simulink model "Longitudinal_Simulink_MaskedParameter_WithOutput_Stateflow"  (Simulink 7.1)
settings: Solver=ode45  StartTime=0.0  StopTime=2.0  RelTol=1e-3
settings Model: Creator=Meisel  LastModifiedBy=Meisel

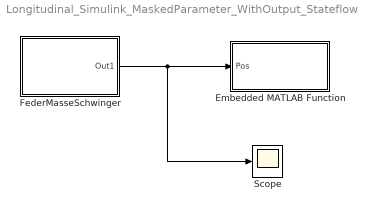
== system Longitudinal_Simulink_MaskedParameter_WithOutput_Stateflow ==
  Embedded MATLAB Function : Stateflow chart
  FederMasseSchwinger : Subsystem  mask{k_init=1000, m=1, l0=1}
      mask prompts: k_init "Federkonstanten"; m "Massen"; l0 "Federlänge"
  Scope : Scope
      settings: TimeRange=0.1792929292929293  YMin=1  YMax=1.888157894736842
  wires:
  FederMasseSchwinger/1(Out1) -> Embedded MATLAB Function/1(Pos), Scope/1

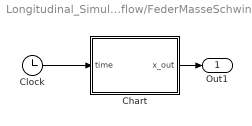
== system Longitudinal_Simulink_MaskedParameter_WithOutput_Stateflow/FederMasseSchwinger ==
  Chart : Stateflow chart
  Clock : Clock
      settings: Decimation=10
  Out1 : Outport
  wires:
  Clock/1 -> Chart/1(time)
  Chart/1(x_out) -> Out1/1

== stateflow chart FederMasseSchwinger/Chart ==
  settings: updateMethod=CONTINUOUS
  state Schwinge
    during:
    // derivatives
    x_dot=v;
    v_dot=Acceleration();
    // output
    x_out=x;
  (default) -> Schwinge : { InitCond(); }
  Schwinge -> Schwinge : [ time >= 0.1 && x0==0 ]
      | { x0=0.4*l0; }
  data: a function_output double size=n; n constant int32 =5; x local double size=n; v local double size=n; k local double size=n; m parameter double; l0 parameter double; time input double; x_out output double size=n; x0 local double; xend local double; k_init parameter double; k0 local double size=1
  data n settings: description=Anzahl der Massen
  data x settings: updateMethod=SF_CONTINUOUS_TIME_DATA  description=Position der Massen
  data v settings: updateMethod=SF_CONTINUOUS_TIME_DATA  description=Geschwindigkeit der Massen
  data k settings: description=Federkonstanten
  data m settings: description=Masse
  data l0 settings: description=Federlänge der entspannten Feder
  data time settings: description=Systemzeit
  data x_out settings: description=Positionen der Massen
  function InitCond:
    | function InitCond
    |     % Die k Massen auf die Startpositionen setzen.
    |     % Abstand zweier Massen: l0
    |     for i = 1:n
    |         x(i) = l0*i;  
    |         k(i) = k_init;
    |     end
    |    
    |     x0   = 0;
    |     k0   = k_init;   % Federkonstante der ersten Feder
    |     xend = double(l0*(n+1));  % warum muss gecastet werden
    | end
  function a  = Acceleration:
    | function a  = Acceleration
    |     
    |     % Size des Rückgabeparameters a muss im 
    |     % ModelExplorer explizit auf n gesetzt werden !!!
    |     a=zeros(n,1);
    |     
    |     % Die erste und die letzte Masse müssen gesondert
    |     % behandelt werden
    |     a(1)=( -(x(1)-x0    -l0)*k0     + (x(2)-x(1)-l0)*k(1) ) / m;
    |     a(n)=( -(x(n)-x(n-1)-l0)*k(n-1) + (xend-x(n)-l0)*k(n) ) / m;    
    |     
    |     % Kraftwirikung zwischen den Massen
    |     for i=2:n-1
    |         a(i) = ( -(x(i)-x(i-1)-l0)*k(i-1) + (x(i+1)-x(i)-l0)*k(i) ) / m;
    |     end
  function Draw:
    | function Draw

== matlab function Embedded MATLAB Function ==
  data: Pos input double
function OutScatter(Pos)
% Embedded MATLAB  

eml.extrinsic('set', 'drawnow', 'scatter', 'gca');
persistent y l0;

    % Init-Parameter
    k  = 5;             % Anzahl der Massen
    l0 = 1;             % Abstand zwischen den Massen
       
    % y-Werte anlegen und mit 0 initialisieren
    y=zeros(1,k);    
   
    % Scatterplot zeichnen
    scatter(Pos', y,  'o', 'MarkerFaceColor', [1 0 0]);
    set (gca,'XLim', [0 (k+1)*l0] );  % x-Bereich festhalten
    drawnow;                          % jetzt zeichnen
end
